simulink model "test"  (R2017a)
settings: Solver=VariableStepAuto  StartTime=0.0  StopTime=10.0  RelTol=1e-3
settings Model: Creator=steven  LastModifiedBy=steven

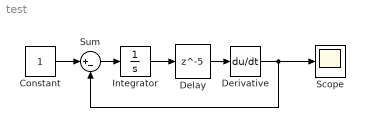
== system test ==
  Constant : Constant
  Delay : Delay  DelayLength=5  InitialCondition=0
  Derivative : Derivative
  Integrator : Integrator
  Scope : Scope
  Sum : Sum  Inputs=|+-
  wires:
  Integrator/1 -> Delay/1
  Derivative/1 -> Scope/1, Sum/2
  Sum/1 -> Integrator/1
  Constant/1 -> Sum/1
  Delay/1 -> Derivative/1
